simulink model "idealIntegrative2DOF"  (R2022b)
settings: Solver=VariableStepAuto  StartTime=0.0  StopTime=Tsim  RelTol=1e-3
values from neighbouring files (symbols this model uses):
  AmpDist = -0.05    [integrativeDTPID.m]
  Tdist = 50    [integrativeDTPID.m]
  Tinit = 0    [integrativeDTPID.m]
libraries: cstblocks x3, simulink x1
settings Model: Creator=jprmj  LastModifiedBy=jprmj

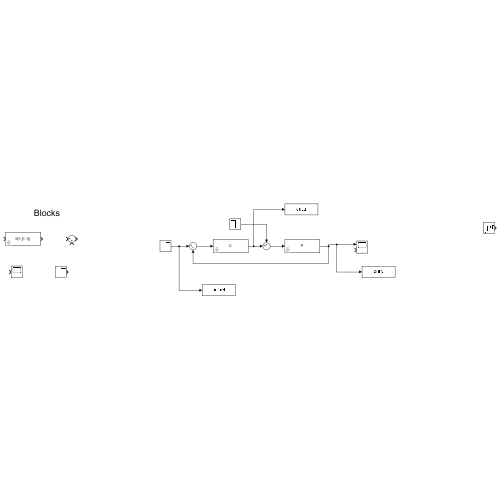
[thumbnail: Simulink's stored preview of the top-level diagram]
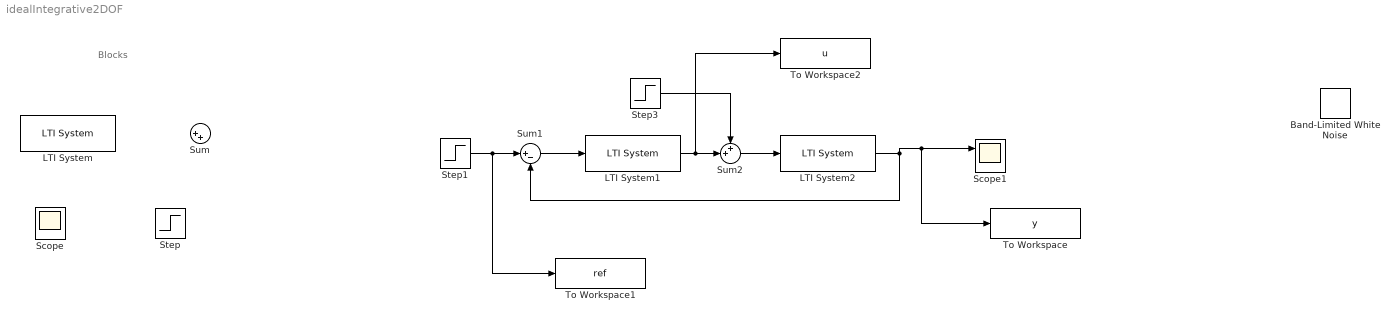
== system idealIntegrative2DOF ==
  note: Blocks
  Band-Limited White Noise : simulink/Sources/Band-Limited White Noise  Cov=[0.1]  Ts=0.1  seed=[23341]
  LTI System : cstblocks/LTI System  sys=tf(1,[1 1])  IC=[]
  LTI System1 : cstblocks/LTI System  sys=C  IC=[]
  LTI System2 : cstblocks/LTI System  sys=P  IC=[]
  Scope : Scope
  Scope1 : Scope  NumInputPorts=2
  Step : Step  SampleTime=0
  Step1 : Step  SampleTime=Tinit
  Step3 : Step  After=AmpDist  SampleTime=Tdist
  Sum : Sum  Inputs=|++
  Sum1 : Sum  Inputs=|+-
  Sum2 : Sum  Inputs=++|
  To Workspace : ToWorkspace  VariableName=y  SaveFormat=Timeseries  SampleTime=-1
  To Workspace1 : ToWorkspace  VariableName=ref  SaveFormat=Timeseries  SampleTime=-1
  To Workspace2 : ToWorkspace  VariableName=u  SaveFormat=Timeseries  SampleTime=-1
  wires:
  LTI System2/1 -> To Workspace/1, Scope1/1, Sum1/2
  Step1/1 -> To Workspace1/1, Sum1/1
  Sum1/1 -> LTI System1/1
  Sum2/1 -> LTI System2/1
  LTI System1/1 -> To Workspace2/1, Sum2/2
  Step3/1 -> Sum2/1
